simulink model "CelciusToFarenheit"  (R2022a)
settings: Solver=VariableStepAuto  StartTime=0.0  StopTime=10.0  RelTol=1e-3
values from neighbouring files (symbols this model uses):
  X = input(prompt)    [CelciusToFarenheitMscript.m]
settings Model: Creator=Waleed  LastModifiedBy=Waleed

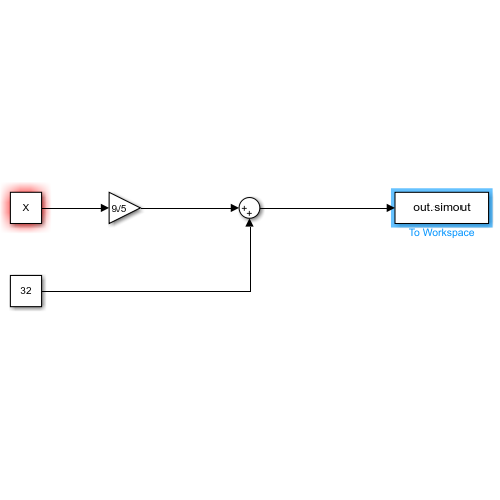
[thumbnail: Simulink's stored preview of the top-level diagram]
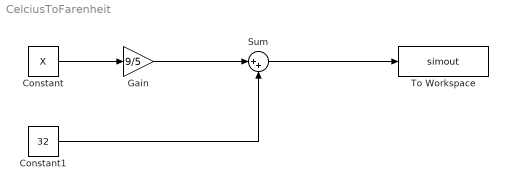
== system CelciusToFarenheit ==
  Constant : Constant  Value=X
  Constant1 : Constant  Value=32
  Gain : Gain  Gain=9/5
  Sum : Sum  Inputs=|++
  To Workspace : ToWorkspace  VariableName=simout  SaveFormat=Timeseries  SampleTime=-1
  wires:
  Constant/1 -> Gain/1
  Gain/1 -> Sum/1
  Constant1/1 -> Sum/2
  Sum/1 -> To Workspace/1
